simulink model "Tutorial_1_sim"  (R2014b)
settings: Solver=ode45  SolverMode=SingleTasking  StartTime=0.0  StopTime=inf  MaxStep=1e-4  RelTol=1e-3
values from neighbouring files (symbols this model uses):
  Ert = 1e3*[unit_params{2}.V, unit_params{3}.V]    [Tutorial_1.m]
  J = 0.0125*Pg/ws    [Tutorial_1.m]
  Kd = 20*J*ws    [Tutorial_1.m]
  Nu = length(subset)    [Tutorial_1.m]
  Pg = 1e6*[unit_params{2}.P, unit_params{3}.P]    [Tutorial_1.m]
  poles = 2    [Tutorial_1.m]
  v1_0 = 0    [Tutorial_1.m]
  v1_d = (2^0.5)*1e3*unit_params{1}.V    [Tutorial_1.m]
  v1_q = 0    [Tutorial_1.m]
  ws = 2*pi*50    (= 314.159265359)    [Tutorial_1.m]
undefined symbols (not defined in the file or in its folder): A, B, C, D, full
settings Model: Creator=COPEC  LastModifiedBy=yoash
settings OptimizationCC: BlockReduction=off  BooleanDataType=off
settings DebuggingCC: SaveWithParameterizedLinksMsg=none  UnderspecifiedInitializationDetection=Classic  MergeDetectMultiDrivingBlocksExec=none  SignalResolutionControl=TryResolveAllWithWarning  SolverPrmCheckMsg=none  FrameProcessingCompatibilityMsg=error
settings HardwareCC: TargetUnknown=on

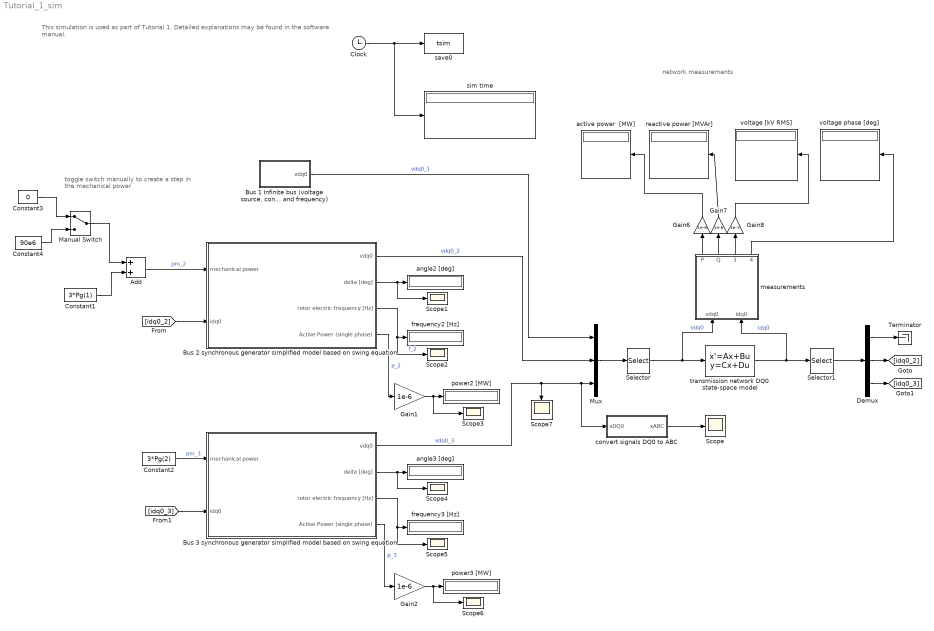
== system Tutorial_1_sim ==
  note: toggle switch manually to
      | create a step in the mechanical power
  note: This simulation is used as part of Tutorial 1.
      |
      | Detailed explanations may be found in the software manual.
  note: network measurements
  Add : Sum
  "Bus 1 Infinite bus (voltage source, constant amplitude and frequency)" : Subsystem
  Bus 2 synchronous generator simplified model based on swing equation : Subsystem
  Bus 3 synchronous generator simplified model based on swing equation : Subsystem
  Clock : Clock
  Constant1 : Constant  Value=3*Pg(1)
  Constant2 : Constant  Value=3*Pg(2)
  Constant3 : Constant  Value=0
  Constant4 : Constant  Value=90e6
  Demux : Demux  Outputs=Nu
  Gain{1..2,6..7} (4 alike) : Gain  Gain=1e-6
  Gain8 : Gain  Gain=1e-3
  Manual Switch : ManualSwitch
  Mux : Mux  Inputs=Nu
  Scope{,1..7} (8 alike) : Scope
      Scope settings: TimeRange=auto  LimitDataPoints=on  MaxDataPoints=5000  SaveToWorkspace=off  SaveName=ScopeData  YMin=-31378.89422  YMax=33665.61525  SampleTime=-1  DataFormat=Array
      Scope1 settings: TimeRange=auto  LimitDataPoints=on  MaxDataPoints=5000  SaveToWorkspace=off  YMin=13.14578396522  YMax=13.14578396553  SampleTime=-1  DataFormat=Array
      Scope2 settings: TimeRange=auto  LimitDataPoints=on  MaxDataPoints=5000  SaveToWorkspace=off  SaveName=ScopeData2  YMin=49.999999999982  YMax=50.000000000009  SampleTime=-1  DataFormat=Array
      Scope3 settings: TimeRange=auto  LimitDataPoints=on  MaxDataPoints=5000  SaveToWorkspace=off  SaveName=ScopeData3  YMin=162.9999999984  YMax=163.0000000004  SampleTime=-1  DataFormat=Array
      Scope4 settings: TimeRange=auto  LimitDataPoints=on  MaxDataPoints=5000  SaveToWorkspace=off  SaveName=ScopeData4  YMin=-10  YMax=10  SampleTime=-1  DataFormat=Array
      Scope5 settings: TimeRange=auto  LimitDataPoints=on  MaxDataPoints=5000  SaveToWorkspace=off  SaveName=ScopeData5  YMin=-10  YMax=10  SampleTime=-1  DataFormat=Array
      Scope6 settings: TimeRange=auto  LimitDataPoints=on  MaxDataPoints=5000  SaveToWorkspace=off  SaveName=ScopeData6  YMin=-10  YMax=10  SampleTime=-1  DataFormat=Array
      Scope7 settings: TimeRange=auto  LimitDataPoints=on  MaxDataPoints=5000  SaveToWorkspace=off  SaveName=ScopeData4  YMin=-3851.36892  YMax=34662.32032  SampleTime=-1  DataFormat=Array
  Selector : Selector  InputPortWidth=3*Nu  IndexOptions=Index vector (dialog)  Indices=units_to_net  OutputSizes=1
  Selector1 : Selector  InputPortWidth=3*Nu  IndexOptions=Index vector (dialog)  Indices=net_to_units  OutputSizes=1
  Terminator : Terminator
  active power  [MW] : Display
  angle2 [deg] : Display
  angle3 [deg] : Display
  "convert signals DQ0 to ABC " : Subsystem
  frequency2 [Hz] : Display
  frequency3 [Hz] : Display
  measurements : Subsystem
  power2 [MW] : Display
  power3 [MW] : Display
  reactive power [MVAr] : Display
  save0 : ToWorkspace  VariableName=tsim  SampleTime=-1
  sim time : Display
  transmission network DQ0 state-space model : StateSpace  A=full(A)  B=full(B)  C=full(C)  D=full(D)  X0=0
  voltage [kV RMS] : Display
  voltage phase [deg] : Display
  wires:
  Clock/1 -> sim time/1, save0/1
  measurements/1(P) -> Gain6/1
  measurements/2(Q) -> Gain7/1
  measurements/3(Vm_RMS) -> Gain8/1
  Gain6/1 -> active power  [MW]/1
  Gain7/1 -> reactive power [MVAr]/1
  Gain8/1 -> voltage [kV RMS]/1
  measurements/4(Vph_deg) -> voltage phase [deg]/1
  Selector/1 -> measurements/1(vdq0), transmission network DQ0 state-space model/1  "vdq0"
  transmission network DQ0 state-space model/1 -> Selector1/1, measurements/2(idq0)  "idq0"
  Mux/1 -> Selector/1
  Selector1/1 -> Demux/1
  Demux/2 -> [idq0_2]
  Demux/3 -> [idq0_3]
  Demux/1 -> Terminator/1
  "convert signals DQ0 to ABC "/1(xABC) -> Scope/1
  "Bus 1 Infinite bus (voltage source, constant amplitude and frequency)"/1(vdq0) -> Mux/1  "vdq0_1"
  Bus 2 synchronous generator simplified model based on swing equation/1(vdq0) -> Mux/2  "vdq0_2"
  [idq0_2] -> Bus 2 synchronous generator simplified model based on swing equation/2(idq0)
  Bus 2 synchronous generator simplified model based on swing equation/2(delta [deg]) -> Scope1/1, angle2 [deg]/1
  Bus 2 synchronous generator simplified model based on swing equation/3(rotor electric frequency [Hz]) -> Scope2/1, frequency2 [Hz]/1  "f_2"
  Bus 3 synchronous generator simplified model based on swing equation/1(vdq0) -> "convert signals DQ0 to ABC "/1(xDQ0), Mux/3, Scope7/1  "vdq0_3"
  [idq0_3] -> Bus 3 synchronous generator simplified model based on swing equation/2(idq0)
  Constant2/1 -> Bus 3 synchronous generator simplified model based on swing equation/1(mechanical power)  "pm_3"
  Bus 3 synchronous generator simplified model based on swing equation/2(delta [deg]) -> Scope4/1, angle3 [deg]/1
  Bus 3 synchronous generator simplified model based on swing equation/3(rotor electric frequency [Hz]) -> Scope5/1, frequency3 [Hz]/1
  Constant1/1 -> Add/2
  Add/1 -> Bus 2 synchronous generator simplified model based on swing equation/1(mechanical power)  "pm_2"
  Manual Switch/1 -> Add/1
  Constant3/1 -> Manual Switch/1
  Constant4/1 -> Manual Switch/2
  Gain1/1 -> Scope3/1, power2 [MW]/1
  Bus 2 synchronous generator simplified model based on swing equation/4(Active Power (single phase)) -> Gain1/1  "p_2"
  Bus 3 synchronous generator simplified model based on swing equation/4(Active Power (single phase)) -> Gain2/1  "p_3"
  Gain2/1 -> Scope6/1, power3 [MW]/1

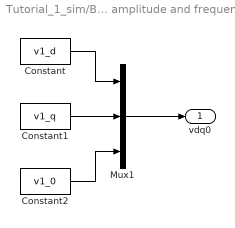
== system Tutorial_1_sim/Bus 1 Infinite bus (voltage source, constant amplitude and frequency) ==
  Constant : Constant  Value=v1_d
  Constant1 : Constant  Value=v1_q
  Constant2 : Constant  Value=v1_0
  Mux1 : Mux  Inputs=3
  vdq0 : Outport
  wires:
  Mux1/1 -> vdq0/1
  Constant/1 -> Mux1/1
  Constant1/1 -> Mux1/2
  Constant2/1 -> Mux1/3

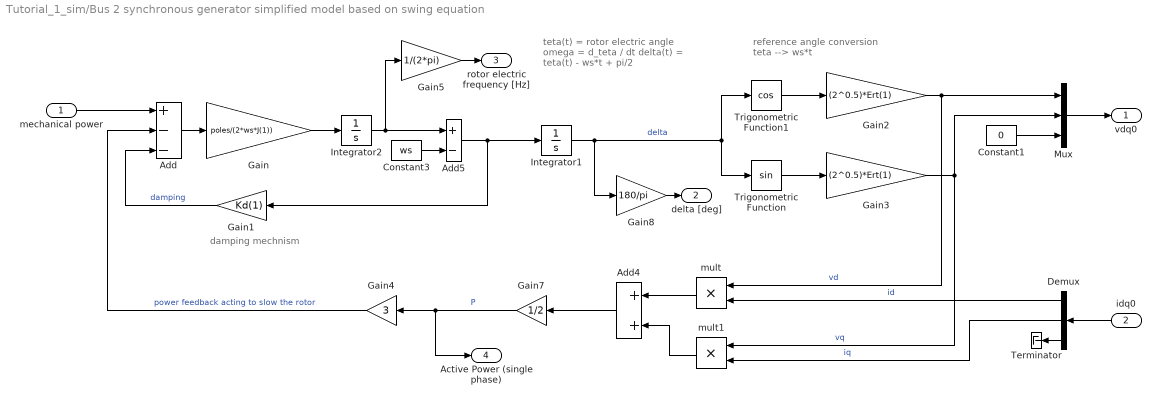
== system Tutorial_1_sim/Bus 2 synchronous generator simplified model based on swing equation ==
  note: reference angle conversion
      | teta --> ws*t
  note: damping mechnism
  note: teta(t) = rotor electric angle
      | omega = d_teta / dt
      | delta(t) = teta(t) - ws*t + pi/2
  mechanical power : Inport
  idq0 : Inport  Port=2
  Add : Sum  Inputs=+--
  Add4 : Sum
  Add5 : Sum  Inputs=+-
  Constant1 : Constant  Value=0
  Constant3 : Constant  Value=ws
  Demux : Demux  Outputs=3
  Gain : Gain  Gain=poles/(2*ws*J(1))
  Gain1 : Gain  Gain=Kd(1)
  Gain2 : Gain  Gain=(2^0.5)*Ert(1)
  Gain3 : Gain  Gain=(2^0.5)*Ert(1)
  Gain4 : Gain  Gain=3
  Gain5 : Gain  Gain=1/(2*pi)
  Gain7 : Gain  Gain=1/2
  Gain8 : Gain  Gain=180/pi
  Integrator1 : Integrator
  Integrator2 : Integrator  InitialCondition=ws
  Mux : Mux  Inputs=3
  Terminator : Terminator
  Trigonometric Function : Trigonometry
  Trigonometric Function1 : Trigonometry  Operator=cos
  mult : Product  Inputs=**
  mult1 : Product  Inputs=**
  vdq0 : Outport
  delta [deg] : Outport  Port=2
  rotor electric frequency [Hz] : Outport  Port=3
  Active Power (single phase) : Outport  Port=4
  wires:
  mechanical power/1 -> Add/1
  Add/1 -> Gain/1
  Gain/1 -> Integrator2/1
  Integrator1/1 -> Gain8/1, Trigonometric Function1/1, Trigonometric Function/1  "delta"
  Gain1/1 -> Add/3  "damping"
  mult/1 -> Add4/1
  mult1/1 -> Add4/2
  Add4/1 -> Gain7/1
  Gain4/1 -> Add/2  "power feedback acting to slow the rotor"
  Gain2/1 -> Mux/1, mult/1  "vd"
  Gain3/1 -> Mux/2, mult1/1  "vq"
  Integrator2/1 -> Add5/1, Gain5/1
  Add5/1 -> Gain1/1, Integrator1/1
  Constant3/1 -> Add5/2
  Trigonometric Function1/1 -> Gain2/1
  Trigonometric Function/1 -> Gain3/1
  Constant1/1 -> Mux/3
  Mux/1 -> vdq0/1
  idq0/1 -> Demux/1
  Demux/1 -> mult/2  "id"
  Demux/2 -> mult1/2  "iq"
  Demux/3 -> Terminator/1
  Gain7/1 -> Active Power (single phase)/1, Gain4/1  "P"
  Gain5/1 -> rotor electric frequency [Hz]/1
  Gain8/1 -> delta [deg]/1

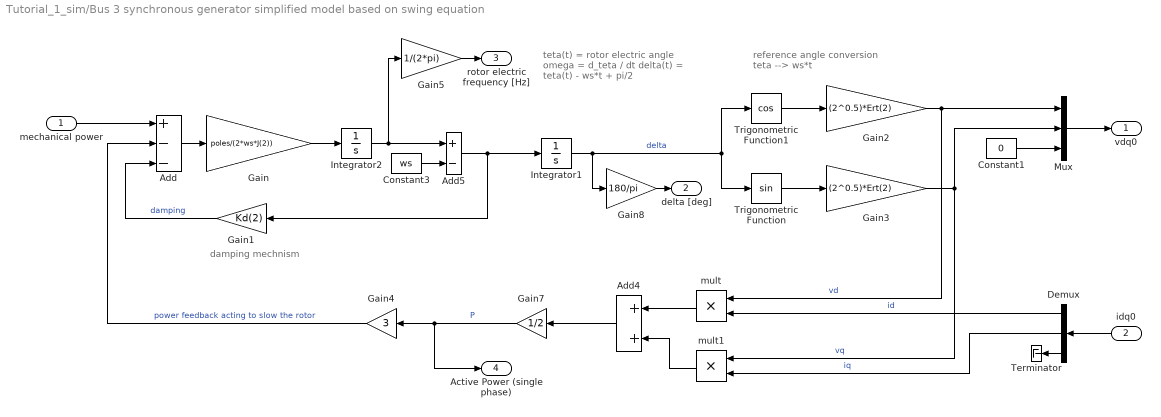
== system Tutorial_1_sim/Bus 3 synchronous generator simplified model based on swing equation ==
  note: reference angle conversion
      | teta --> ws*t
  note: damping mechnism
  note: teta(t) = rotor electric angle
      | omega = d_teta / dt
      | delta(t) = teta(t) - ws*t + pi/2
  mechanical power : Inport
  idq0 : Inport  Port=2
  Add : Sum  Inputs=+--
  Add4 : Sum
  Add5 : Sum  Inputs=+-
  Constant1 : Constant  Value=0
  Constant3 : Constant  Value=ws
  Demux : Demux  Outputs=3
  Gain : Gain  Gain=poles/(2*ws*J(2))
  Gain1 : Gain  Gain=Kd(2)
  Gain2 : Gain  Gain=(2^0.5)*Ert(2)
  Gain3 : Gain  Gain=(2^0.5)*Ert(2)
  Gain4 : Gain  Gain=3
  Gain5 : Gain  Gain=1/(2*pi)
  Gain7 : Gain  Gain=1/2
  Gain8 : Gain  Gain=180/pi
  Integrator1 : Integrator
  Integrator2 : Integrator  InitialCondition=ws
  Mux : Mux  Inputs=3
  Terminator : Terminator
  Trigonometric Function : Trigonometry
  Trigonometric Function1 : Trigonometry  Operator=cos
  mult : Product  Inputs=**
  mult1 : Product  Inputs=**
  vdq0 : Outport
  delta [deg] : Outport  Port=2
  rotor electric frequency [Hz] : Outport  Port=3
  Active Power (single phase) : Outport  Port=4
  wires:
  mechanical power/1 -> Add/1
  Add/1 -> Gain/1
  Gain/1 -> Integrator2/1
  Integrator1/1 -> Gain8/1, Trigonometric Function1/1, Trigonometric Function/1  "delta"
  Gain1/1 -> Add/3  "damping"
  mult/1 -> Add4/1
  mult1/1 -> Add4/2
  Add4/1 -> Gain7/1
  Gain4/1 -> Add/2  "power feedback acting to slow the rotor"
  Gain2/1 -> Mux/1, mult/1  "vd"
  Gain3/1 -> Mux/2, mult1/1  "vq"
  Integrator2/1 -> Gain5/1, Add5/1
  Add5/1 -> Gain1/1, Integrator1/1
  Constant3/1 -> Add5/2
  Trigonometric Function1/1 -> Gain2/1
  Trigonometric Function/1 -> Gain3/1
  Constant1/1 -> Mux/3
  Mux/1 -> vdq0/1
  idq0/1 -> Demux/1
  Demux/1 -> mult/2  "id"
  Demux/2 -> mult1/2  "iq"
  Demux/3 -> Terminator/1
  Gain7/1 -> Active Power (single phase)/1, Gain4/1  "P"
  Gain5/1 -> rotor electric frequency [Hz]/1
  Gain8/1 -> delta [deg]/1

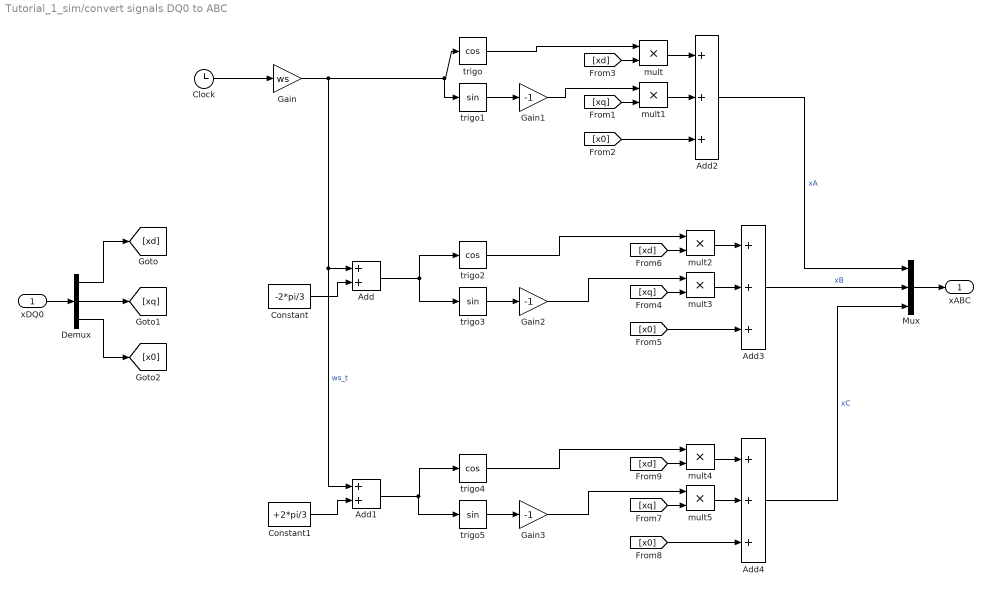
== system Tutorial_1_sim/convert signals DQ0 to ABC  ==
  xDQ0 : Inport
  Add : Sum
  Add1 : Sum
  Add2 : Sum  Inputs=+++
  Add3 : Sum  Inputs=+++
  Add4 : Sum  Inputs=+++
  Clock : Clock
  Constant : Constant  Value=-2*pi/3
  Constant1 : Constant  Value=+2*pi/3
  Demux : Demux  Outputs=3
  Gain : Gain  Gain=ws
  Gain1 : Gain  Gain=-1
  Gain2 : Gain  Gain=-1
  Gain3 : Gain  Gain=-1
  Mux : Mux  Inputs=3
  mult{,1..5} (6 alike) : Product  Inputs=**
  trigo : Trigonometry  Operator=cos
  trigo1 : Trigonometry
  trigo2 : Trigonometry  Operator=cos
  trigo3 : Trigonometry
  trigo4 : Trigonometry  Operator=cos
  trigo5 : Trigonometry
  xABC : Outport
  wires:
  Clock/1 -> Gain/1
  Gain/1 -> trigo1/1, trigo/1, Add1/1, Add/1  "ws_t"
  Constant/1 -> Add/2
  Constant1/1 -> Add1/2
  trigo1/1 -> Gain1/1
  trigo3/1 -> Gain2/1
  Add/1 -> trigo2/1, trigo3/1
  trigo5/1 -> Gain3/1
  Add1/1 -> trigo5/1, trigo4/1
  xDQ0/1 -> Demux/1
  Demux/1 -> [xd]
  Demux/2 -> [xq]
  Demux/3 -> [x0]
  Mux/1 -> xABC/1
  mult/1 -> Add2/1
  mult1/1 -> Add2/2
  [xd] -> mult/2
  [xq] -> mult1/2
  [x0] -> Add2/3
  mult2/1 -> Add3/1
  mult3/1 -> Add3/2
  [xd] -> mult2/2
  [xq] -> mult3/2
  [x0] -> Add3/3
  mult4/1 -> Add4/1
  mult5/1 -> Add4/2
  [xd] -> mult4/2
  [xq] -> mult5/2
  [x0] -> Add4/3
  trigo/1 -> mult/1
  Gain1/1 -> mult1/1
  trigo2/1 -> mult2/1
  Gain2/1 -> mult3/1
  trigo4/1 -> mult4/1
  Gain3/1 -> mult5/1
  Add2/1 -> Mux/1  "xA"
  Add3/1 -> Mux/2  "xB"
  Add4/1 -> Mux/3  "xC"

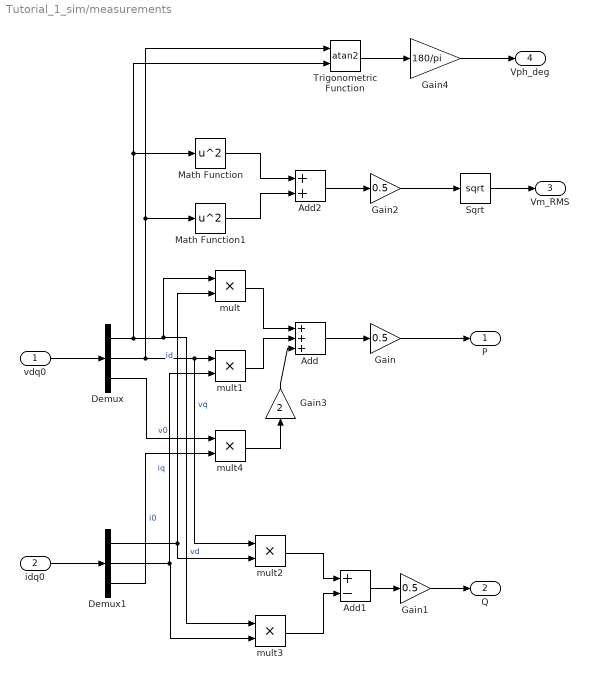
== system Tutorial_1_sim/measurements ==
  vdq0 : Inport
  idq0 : Inport  Port=2
  Add : Sum  Inputs=+++
  Add1 : Sum  Inputs=+-
  Add2 : Sum
  Demux : Demux  Outputs=3
  Demux1 : Demux  Outputs=3
  Gain : Gain  Gain=0.5
  Gain1 : Gain  Gain=0.5
  Gain2 : Gain  Gain=0.5
  Gain3 : Gain  Gain=2
  Gain4 : Gain  Gain=180/pi
  Math Function : Math  Operator=square  SaturateOnIntegerOverflow=on
  Math Function1 : Math  Operator=square  SaturateOnIntegerOverflow=on
  Sqrt : Sqrt  SaturateOnIntegerOverflow=on
  Trigonometric Function : Trigonometry  Operator=atan2
  mult{,1..4} (5 alike) : Product  Inputs=**
  P : Outport
  Q : Outport  Port=2
  Vm_RMS : Outport  Port=3
  Vph_deg : Outport  Port=4
  wires:
  idq0/1 -> Demux1/1
  vdq0/1 -> Demux/1
  Demux/1 -> Math Function/1, Trigonometric Function/2, mult3/1, mult/1  "vd"
  Demux/2 -> Trigonometric Function/1, Math Function1/1, mult2/1, mult1/1  "vq"
  Demux1/1 -> mult/2, mult2/2  "id"
  Demux1/2 -> mult3/2, mult1/2  "iq"
  Demux/3 -> mult4/1  "v0"
  Demux1/3 -> mult4/2  "i0"
  mult/1 -> Add/1
  mult1/1 -> Add/2
  Add/1 -> Gain/1
  mult2/1 -> Add1/1
  mult3/1 -> Add1/2
  Add1/1 -> Gain1/1
  Sqrt/1 -> Vm_RMS/1
  Math Function/1 -> Add2/1
  Math Function1/1 -> Add2/2
  Add2/1 -> Gain2/1
  Gain2/1 -> Sqrt/1
  Gain/1 -> P/1
  Gain1/1 -> Q/1
  mult4/1 -> Gain3/1
  Gain3/1 -> Add/3
  Trigonometric Function/1 -> Gain4/1
  Gain4/1 -> Vph_deg/1
